simulink model "controle_malha_fechada"  (R2021a)
settings: Solver=VariableStepAuto  StartTime=0.0  StopTime=2.0  RelTol=1e-3
settings Model: Creator=caioc  LastModifiedBy=caioc

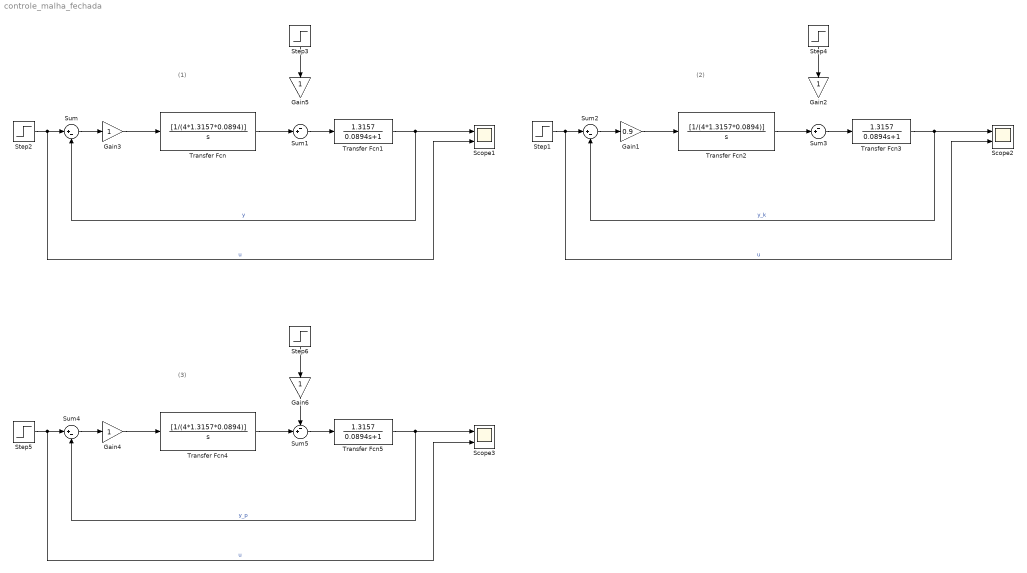
== system controle_malha_fechada ==
  note: (1)
  note: (2)
  note: (3)
  Gain1 : Gain  Gain=0.9
  Gain{2..6} (5 alike) : Gain
  Scope1 : Scope  NumInputPorts=2
  Scope2 : Scope  NumInputPorts=2
  Scope3 : Scope  NumInputPorts=2
  Step1 : Step  Time=0  After=10  SampleTime=0
  Step2 : Step  Time=0  After=10  SampleTime=0
  Step3 : Step  Time=0  After=0.45  SampleTime=0
  Step4 : Step  Time=0  After=0.45  SampleTime=0
  Step5 : Step  Time=0  After=10  SampleTime=0
  Step6 : Step  Time=0  After=0.45  SampleTime=0
  Sum : Sum  Inputs=|+-
  Sum1 : Sum  Inputs=-+|
  Sum2 : Sum  Inputs=|+-
  Sum3 : Sum  Inputs=-+|
  Sum4 : Sum  Inputs=|+-
  Sum5 : Sum  Inputs=-+|
  Transfer Fcn : TransferFcn  Numerator=[1/(4*1.3157*0.0894)]  Denominator=[1 0]
  Transfer Fcn1 : TransferFcn  Numerator=[1.3157]  Denominator=[0.0894 1]
  Transfer Fcn2 : TransferFcn  Numerator=[1/(4*1.3157*0.0894)]  Denominator=[1 0]
  Transfer Fcn3 : TransferFcn  Numerator=[1.3157]  Denominator=[0.0894 1]
  Transfer Fcn4 : TransferFcn  Numerator=[1/(4*1.3157*0.0894)]  Denominator=[1 0]
  Transfer Fcn5 : TransferFcn  Numerator=[1.3157]  Denominator=[0.0894 1]
  wires:
  Gain3/1 -> Transfer Fcn/1
  Transfer Fcn1/1 -> Sum/2, Scope1/1  "y"
  Sum1/1 -> Transfer Fcn1/1
  Step3/1 -> Gain5/1
  Step2/1 -> Sum/1, Scope1/2  "u"
  Transfer Fcn/1 -> Sum1/2
  Sum/1 -> Gain3/1
  Sum2/1 -> Gain1/1
  Step4/1 -> Gain2/1
  Step1/1 -> Sum2/1, Scope2/2  "u"
  Sum3/1 -> Transfer Fcn3/1
  Transfer Fcn3/1 -> Sum2/2, Scope2/1  "y_k"
  Gain1/1 -> Transfer Fcn2/1
  Transfer Fcn2/1 -> Sum3/2
  Sum4/1 -> Gain4/1
  Step6/1 -> Gain6/1
  Step5/1 -> Sum4/1, Scope3/2  "u"
  Sum5/1 -> Transfer Fcn5/1
  Transfer Fcn5/1 -> Sum4/2, Scope3/1  "y_p"
  Gain4/1 -> Transfer Fcn4/1
  Transfer Fcn4/1 -> Sum5/2
  Gain6/1 -> Sum5/1
